simulink model "CM515A_MotAg4Meas"  (R2013b)
settings: Solver=VariableStepDiscrete  SolverMode=SingleTasking  StartTime=0.0  StopTime=1  FixedStep=0.002  RelTol=1e-3
values from neighbouring files (symbols this model uses):
  MOTAGCNTRREGMASK_CNT_U16 = DataDict.Constant    [CM515A_MotAg4Meas_DataDict.m]
  MOTAGLIM_CNT_U16 = DataDict.Constant    [CM515A_MotAg4Meas_DataDict.m]
undefined symbols (not defined in the file or in its folder): sigbuilder_block
libraries: simulink x4, NexteerUtilities x1
settings Model: RequirementInfo="{}  %GIDa_ca294f38_ed7c_4fb9_8c54_f4d56271bfc7"  ModifiedHistory=Rev 008: Updated model to Matlab 2013B, added comments to show requirement linkage  PauseTimes=0.5  Creator=nz3zln  LastModifiedBy=tzbsjd
settings SolverCC: AutoInsertRateTranBlk=on  InsertRTBMode=Always
settings DataIOCC: LimitDataPoints=off  SaveFormat=Structure  ReturnWorkspaceOutputs=on
settings OptimizationCC: BlockReduction=off  InlineParams=on  ZeroExternalMemoryAtStartup=off  ZeroInternalMemoryAtStartup=off  OptimizeModelRefInitCode=on  LifeSpan=1
settings DebuggingCC: SignalInfNanChecking=error  SignalRangeChecking=warning  UnderspecifiedInitializationDetection=Simplified  SolverPrmCheckMsg=error  InheritedTsInSrcMsg=error  DiscreteInheritContinuousMsg=error  SingleTaskRateTransMsg=error  TasksWithSamePriorityMsg=error  SigSpecEnsureSampleTimeMsg=error  CheckMatrixSingularityMsg=error  ParameterUnderflowMsg=error  ParameterPrecisionLossMsg=error  ParameterTunabilityLossMsg=error  FixptConstUnderflowMsg=warning  FixptConstOverflowMsg=warning  VectorMatrixConversionMsg=error  SignalLabelMismatchMsg=error  UnconnectedInputMsg=error  UnconnectedOutputMsg=error  UnconnectedLineMsg=error  SFcnCompatibilityMsg=error  UniqueDataStoreMsg=warning  BusObjectLabelMismatch=error  RootOutportRequireBusObject=error  AssertControl=DisableAll  ModelReferenceIOMsg=error  ModelReferenceVersionMismatchMessage=warning  ModelReferenceIOMismatchMessage=error  ModelReferenceCSMismatchMessage=warning  ModelReferenceDataLoggingMessage=error  StateNameClashWarn=warning  StrictBusMsg=ErrorOnBusTreatedAsVector  NonBusSignalsTreatedAsBus=error  SFUnexpectedBacktrackingDiag=error  SFInvalidInputDataAccessInChartInitDiag=error  SFNoUnconditionalDefaultTransitionDiag=error  SFTransitionOutsideNaturalParentDiag=error  SFUnconditionalTransitionShadowingDiag=error  SFUndirectedBroadcastEventsDiag=error
settings ModelReferenceCC: ModelReferenceNumInstancesAllowed=Single
settings RTWCC: SystemTargetFile=autosar.tlc  GenCodeOnly=on  TemplateMakefile=ert_default_tmf  Description=AUTOSAR  GenerateReport=on  ProcessScript=autosar_make_rtw_hook  LaunchReport=on
settings CodeAppCC: GenerateComments=off  IgnoreCustomStorageClasses=off  CustomSymbolStrType=$N$R$M  CustomSymbolStrBlkIO=$N$M  SimulinkBlockComments=off
settings STFCustomTargetCC: ParMdlRefBuildCompliant=on  CompOptLevelCompliant=on  IncludeMdlTerminateFcn=off  CombineOutputUpdateFcns=on  SuppressErrorStatus=on  ERTFirstTimeCompliant=on  ERTCustomFileBanners=on  SupportNonFinite=off  SupportComplex=off  SupportContinuousTime=off  SupportNonInlinedSFcns=off  MATLABClassNameForMDSCustomization=Simulink.SoftwareTarget.ERTCustomization  AutosarCompliant=on  GRTInterface=off  SystemTargetFile=autosar.tlc
settings ERTTargetCC: CodeReplacementLibrary=ANSI_C  ConcurrentExecutionCompliant=off  IncludeMdlTerminateFcn=off  SuppressErrorStatus=on  SupportNonFinite=off  SupportComplex=off  ModelStepFunctionPrototypeControlCompliant=off  CPPClassGenCompliant=off  AutosarCompliant=on  InlinedParameterPlacement=NonHierarchical  ERTCustomFileTemplate=example_file_process.tlc  EnableUserReplacementTypes=on

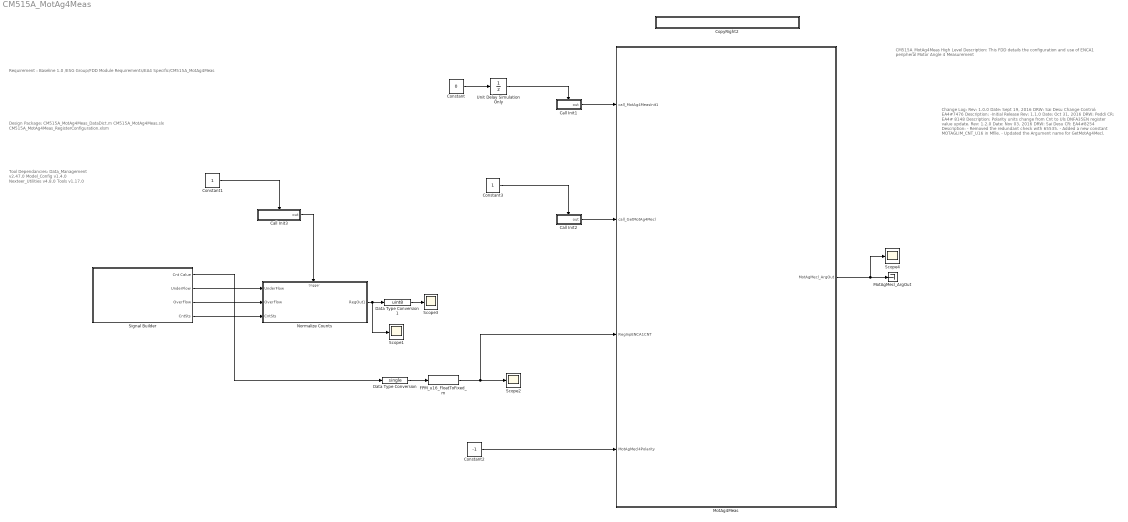
== system CM515A_MotAg4Meas ==
  note: Requirement : Baseline 1.0
      | /ESG Group/FDD Module Requirements/EA4 Specific/CM515A_MotAg4Meas
  note: Design Package:
      | CM515A_MotAg4Meas_DataDict.m
      | CM515A_MotAg4Meas.slx
      | CM515A_MotAg4Meas_RegisterConfiguration.xlsm
  note: CM515A_MotAg4Meas
      | High Level Description:
      | This FDD details the configuration and use of ENCA1 peripheral Motor Angle 4 Measurement
  note: Tool Dependancies:
      | Data_Management v2.47.0
      | Model_Config v1.4.0
      | Nexteer_Utilities v4.8.0
      | Tools v1.17.0
  note: Change Log:
      |
      | Rev: 1.0.0
      | Date: Sept 19, 2016
      | DRW: Sai Desu
      | Change Control: EA4#7476
      | Description:
      | -Initial Release
      |
      | Rev: 1.1.0
      | Date: Oct 31, 2016
      | DRW: Peddi
      | CR: EA4# 8148
      | Description: Polarity units change from Cnt to Uls
      | DNFA35EN register value update.
      |
      | Rev: 1.2.0
      | Date: Nov 03, 2016
      | DRW: Sai Desu
      | CR: EA4#8254
      | Description:
      | - Removed the redundant check with 65535.
      | - Added a new constant MOTAGLIM_CNT_U16 in  Mfile.
      | - Updated the Argument name for GetMotAg4Mecl.
  Call Init1 : Subsystem  TreatAsAtomicUnit=on
  Call Init2 : Subsystem  TreatAsAtomicUnit=on
  Call Init3 : Subsystem  TreatAsAtomicUnit=on
  Constant : Constant  Value=0  OutDataTypeStr=uint8
  Constant1 : Constant  OutDataTypeStr=int8
  Constant2 : Constant  Value=-1  OutDataTypeStr=int8
  Constant3 : Constant  OutDataTypeStr=int8
  CopyRight2 : Subsystem  Description=|  mask(Copyright Information){none=on}
      | Copyright info block.                                               
      |                                                                     
      | Place copyright information at the top of every subsystem in design.
      mask prompts: none "No parameters"
      mask help: Place copyright information at the top of every subsystem in design.
      mask Display:
      | NxtrConf = 'Nexteer Confidential';
      | 
      | sys = bdroot; %handle for the current model ("system")
      | first = get_param(sys,'Created');
      | first = first(end-3:end);  %year is last four digits
      | 
      | last = get_param(sys,'LastModifiedDate');
      | if isempty(last)
      |     last = datestr(now,'yyyy');
      | else
      |     last = last(end-3:end);
      | end
      | 
      | if strcmp(first,last)
      |     fprintf('%s -- Copyright %s Nexteer',NxtrConf,first)
      | else
      |     fprintf('%s -- %s%s- %s Nexteer',NxtrConf,char(169),first,last)
      | end
  Data Type Conversion : DataTypeConversion  OutDataTypeStr=single
  Data Type Conversion1 : DataTypeConversion  OutDataTypeStr=uint8
  FPM_u16_FloatToFixed_m : NexteerUtilities/Fixed Point Math Conversions/FPM_u16_FloatToFixed_m  SFunctionSpec=uint16 y1 = FPM_u16_FloatToFixed_m(single u1, single p1)  Param1=16
      settings: AttributesFormatString=u16_FloatToFixed
  MotAg4Meas : Subsystem
  MotAgMecl_ArgOut : Terminator
  Normalize Counts : Subsystem
  Scope{1..4} (4 alike) : Scope
      Scope2 settings: SaveName=ScopeData7
      Scope4 settings: SaveName=ScopeData2
  Signal Builder : Subsystem  Tag=STV Subsys  LoadFcn=sigbuilder_block('load');  StartFcn=sigbuilder_block('start');  StopFcn=sigbuilder_block('stop');  ClipboardFcn=sigbuilder_block('clipboard');  mask(Sigbuilder block){}
      mask help: Simulink:masks:SigbuilderBlock_MD
      mask init:
      | if ~strcmp(get_param(bdroot(gcbh),'SimulationStatus'),'stopped') tuvar = sigbuilder_block('maskInit'); end
      settings: CopyFcn=sigbuilder_block('copy');  DeleteFcn=sigbuilder_block('delete');  ModelCloseFcn=sigbuilder_block('modelClose');  PreSaveFcn=sigbuilder_block('preSave');  PauseFcn=sigbuilder_block('pause');  ContinueFcn=sigbuilder_block('continue');  NameChangeFcn=sigbuilder_block('namechange');  OpenFcn=sigbuilder_block('open',[0 30 1440 723 ]);  CloseFcn=sigbuilder_block('close');
      mask Display: plot(0, 0, 100, 100,[2, 2, 32, 32, 2], [68, 8, 8, 68, 68],[32, 2], [38, 38], [32, 19, 2],[53, 60, 44], [32, 17, 17, 2],[16, 16, 31, 31]);txt = getActiveGroup(gcbh);text(2, 100, txt,'verticalAlignment', 'top');
  Unit Delay Simulation Only : UnitDelay  InitialCondition=1  SampleTime=-1
  wires:
  Constant/1 -> Unit Delay Simulation Only/1
  Unit Delay Simulation Only/1 -> Call Init1/Enable
  Constant3/1 -> Call Init2/Enable
  Call Init1/1(out) -> MotAg4Meas/1(call_MotAg4MeasInit1)
  Call Init2/1(out) -> MotAg4Meas/2(call_GetMotAg4Mecl)
  FPM_u16_FloatToFixed_m/1 -> MotAg4Meas/3(RegInpENCA1CNT), Scope2/1
  Normalize Counts/1(RegOut1) -> Data Type Conversion1/1, Scope1/1
  MotAg4Meas/1(MotAgMecl_ArgOut) -> Scope4/1, MotAgMecl_ArgOut/1
  Data Type Conversion/1 -> FPM_u16_FloatToFixed_m/1
  Constant1/1 -> Call Init3/Enable
  Call Init3/1(out) -> Normalize Counts/Trigger
  Signal Builder/1(Cnt Calue) -> Data Type Conversion/1
  Signal Builder/2(UnderFlow) -> Normalize Counts/1(UnderFlow)
  Signal Builder/3(OverFlow) -> Normalize Counts/2(OverFlow)
  Signal Builder/4(CntSts) -> Normalize Counts/3(CntSts)
  Data Type Conversion1/1 -> Scope3/1
  Constant2/1 -> MotAg4Meas/4(MotAgMecl4Polarity)

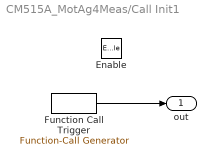
== system CM515A_MotAg4Meas/Call Init1 ==
  Enable : EnablePort
  Function Call Trigger : simulink/Ports & Subsystems/Function-Call Generator  RequirementInfo={} %GIDa_b7229461_487a_40de_bfdf_dab388053d82  sample_time=0.002  numberOfIterations=1
  out : Outport
  wires:
  Function Call Trigger/1 -> out/1

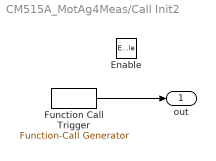
== system CM515A_MotAg4Meas/Call Init2 ==
  Enable : EnablePort
  Function Call Trigger : simulink/Ports & Subsystems/Function-Call Generator  RequirementInfo={} %GIDa_a0a97c4f_3e8f_431b_a781_191ff84f73ef  sample_time=0.0005  numberOfIterations=1
  out : Outport
  wires:
  Function Call Trigger/1 -> out/1

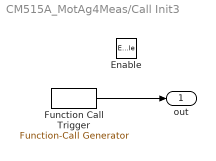
== system CM515A_MotAg4Meas/Call Init3 ==
  Enable : EnablePort
  Function Call Trigger : simulink/Ports & Subsystems/Function-Call Generator  RequirementInfo={} %GIDa_a0a97c4f_3e8f_431b_a781_191ff84f73ef  sample_time=0.0005  numberOfIterations=1
  out : Outport
  wires:
  Function Call Trigger/1 -> out/1

== system CM515A_MotAg4Meas/CopyRight2 ==

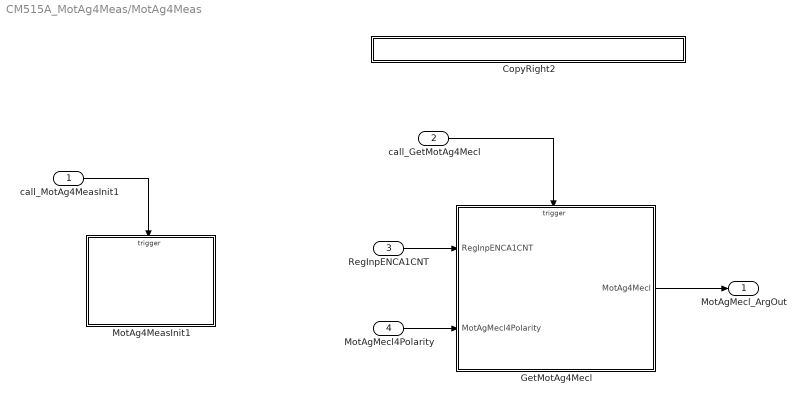
== system CM515A_MotAg4Meas/MotAg4Meas ==
  call_MotAg4MeasInit1 : Inport  RequirementInfo={} %GIDa_3f2124e9_01f6_42c8_98ca_c09f4c17d99d
  call_GetMotAg4Mecl : Inport  RequirementInfo={} %GIDa_a9829b41_47bf_4b01_8e96_1bb4faec4565  Port=2
  RegInpENCA1CNT : Inport  Port=3
  MotAgMecl4Polarity : Inport  Port=4
  CopyRight2 : Subsystem  Description=|  mask(Copyright Information){none=on}
      | Copyright info block.                                               
      |                                                                     
      | Place copyright information at the top of every subsystem in design.
      mask prompts: none "No parameters"
      mask help: Place copyright information at the top of every subsystem in design.
      mask Display:
      | NxtrConf = 'Nexteer Confidential';
      | 
      | sys = bdroot; %handle for the current model ("system")
      | first = get_param(sys,'Created');
      | first = first(end-3:end);  %year is last four digits
      | 
      | last = get_param(sys,'LastModifiedDate');
      | if isempty(last)
      |     last = datestr(now,'yyyy');
      | else
      |     last = last(end-3:end);
      | end
      | 
      | if strcmp(first,last)
      |     fprintf('%s -- Copyright %s Nexteer',NxtrConf,first)
      | else
      |     fprintf('%s -- %s%s- %s Nexteer',NxtrConf,char(169),first,last)
      | end
  GetMotAg4Mecl : Subsystem  RequirementInfo={} %GIDa_dbd08618_b447_4b13_a314_37af3685d10a
  MotAg4MeasInit1 : Subsystem
  MotAgMecl_ArgOut : Outport
  wires:
  call_MotAg4MeasInit1/1 -> MotAg4MeasInit1/Trigger
  call_GetMotAg4Mecl/1 -> GetMotAg4Mecl/Trigger
  RegInpENCA1CNT/1 -> GetMotAg4Mecl/1(RegInpENCA1CNT)
  GetMotAg4Mecl/1(MotAg4Mecl) -> MotAgMecl_ArgOut/1
  MotAgMecl4Polarity/1 -> GetMotAg4Mecl/2(MotAgMecl4Polarity)

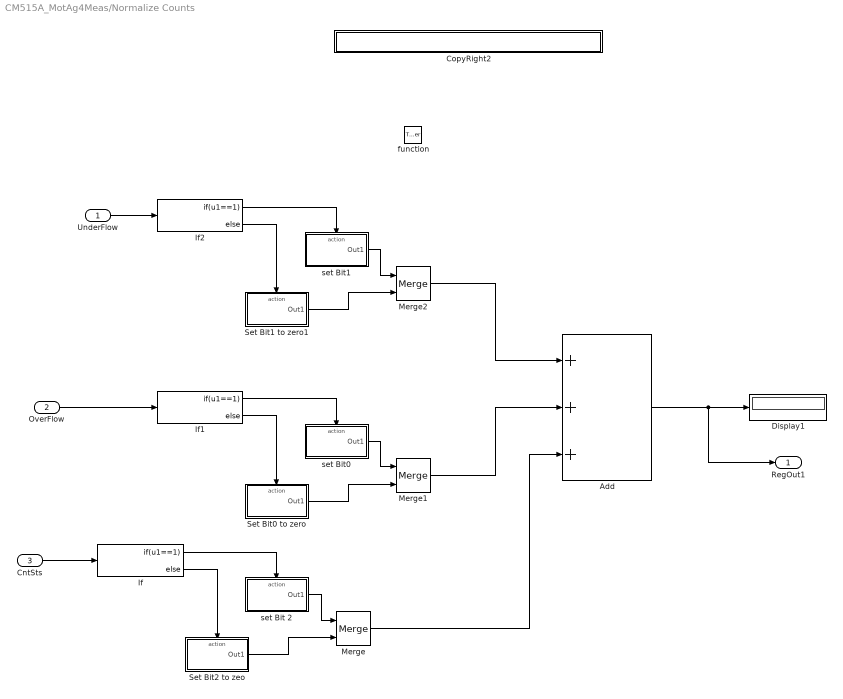
== system CM515A_MotAg4Meas/Normalize Counts ==
  UnderFlow : Inport
  OverFlow : Inport  Port=2
  CntSts : Inport  Port=3
  function : TriggerPort  TriggerType=function-call
  Add : Sum  Inputs=+++
  CopyRight2 : Subsystem  Description=|  mask(Copyright Information){none=on}
      | Copyright info block.                                               
      |                                                                     
      | Place copyright information at the top of every subsystem in design.
      mask prompts: none "No parameters"
      mask help: Place copyright information at the top of every subsystem in design.
      mask Display:
      | NxtrConf = 'Nexteer Confidential';
      | 
      | sys = bdroot; %handle for the current model ("system")
      | first = get_param(sys,'Created');
      | first = first(end-3:end);  %year is last four digits
      | 
      | last = get_param(sys,'LastModifiedDate');
      | if isempty(last)
      |     last = datestr(now,'yyyy');
      | else
      |     last = last(end-3:end);
      | end
      | 
      | if strcmp(first,last)
      |     fprintf('%s -- Copyright %s Nexteer',NxtrConf,first)
      | else
      |     fprintf('%s -- %s%s- %s Nexteer',NxtrConf,char(169),first,last)
      | end
  Display1 : Display
  If : If  IfExpression=u1==1
  If1 : If  IfExpression=u1==1
  If2 : If  IfExpression=u1==1
  Merge : Merge
  Merge1 : Merge
  Merge2 : Merge
  Set Bit0 to zero : Subsystem  TreatAsAtomicUnit=on
  Set Bit1 to zero1 : Subsystem  TreatAsAtomicUnit=on
  Set Bit2 to zeo : Subsystem  TreatAsAtomicUnit=on
  set Bit 2 : Subsystem  TreatAsAtomicUnit=on
  set Bit0 : Subsystem  TreatAsAtomicUnit=on
  set Bit1 : Subsystem  TreatAsAtomicUnit=on
  RegOut1 : Outport
  wires:
  CntSts/1 -> If/1
  If/1 -> set Bit 2/Action
  If/2 -> Set Bit2 to zeo/Action
  set Bit 2/1(Out1) -> Merge/1
  Set Bit2 to zeo/1(Out1) -> Merge/2
  If1/1 -> set Bit0/Action
  If1/2 -> Set Bit0 to zero/Action
  set Bit0/1(Out1) -> Merge1/1
  Set Bit0 to zero/1(Out1) -> Merge1/2
  OverFlow/1 -> If1/1
  If2/1 -> set Bit1/Action
  If2/2 -> Set Bit1 to zero1/Action
  set Bit1/1(Out1) -> Merge2/1
  Set Bit1 to zero1/1(Out1) -> Merge2/2
  UnderFlow/1 -> If2/1
  Merge2/1 -> Add/1
  Merge1/1 -> Add/2
  Merge/1 -> Add/3
  Add/1 -> RegOut1/1, Display1/1

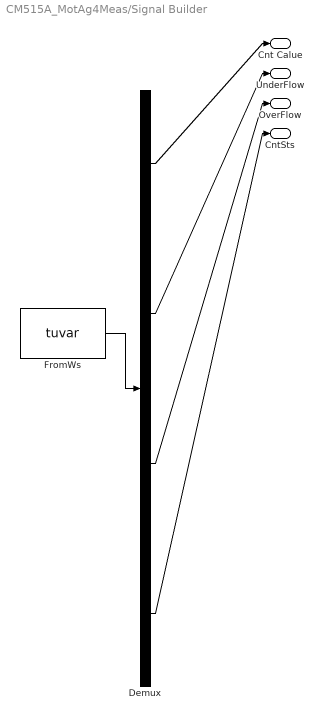
== system CM515A_MotAg4Meas/Signal Builder ==
  Demux : Demux  Tag=STV Demux
  FromWs : FromWorkspace  Tag=STV FromWs  VariableName=tuvar  SampleTime=0
      SigBuilderData=|
      | common.afterFinalStr = 'Extrapolate'
      | common.sampleTime = 0
      | dataSet(1).timeRange = [0 1]
      | dataSet(1).name = 'UpCount'
      | dataSet(2).timeRange = [0 1]
      | dataSet(2).name = 'DownCount'
      | sbobj.Groups(1).Name = 'UpCount'
      | sbobj.Groups(1).Signals(1).Name = 'Cnt Calue'
      | sbobj.Groups(1).Signals(1).XData = [0 0.2 0.2 0.3 0.4 0.4 0.6 1]
      | sbobj.Groups(1).Signals(1).YData = [0 1 0 0.5 0 1 0 1]
      | sbobj.Groups(1).Signals(2).Name = 'UnderFlow'
      | sbobj.Groups(1).Signals(2).XData = [0 0.5 1]
      | sbobj.Groups(1).Signals(2).YData = [0 0 0]
      | sbobj.Groups(1).Signals(3).Name = 'OverFlow'
      | sbobj.Groups(1).Signals(3).XData = [0 0.499 0.499 0.5 0.5 1]
      | sbobj.Groups(1).Signals(3).YData = [0 0 1 1 0 0]
      | sbobj.Groups(1).Signals(4).Name = 'CntSts'
      | sbobj.Groups(1).Signals(4).XData = [0 1]
      | sbobj.Groups(1).Signals(4).YData = [0 0]
      | sbobj.Groups(1).TimeRange = [0 1]
      | sbobj.Groups(2).Name = 'DownCount'
      | sbobj.Groups(2).Signals(1).Name = 'Cnt Calue'
      | sbobj.Groups(2).Signals(1).XData = [0 1]
      | sbobj.Groups(2).Signals(1).YData = [1 0]
      | sbobj.Groups(2).Signals(2).Name = 'UnderFlow'
      | sbobj.Groups(2).Signals(2).XData = [0 0.499 0.499 0.5 0.5 1]
      | sbobj.Groups(2).Signals(2).YData = [0 0 1 1 0 0]
      | sbobj.Groups(2).Signals(3).Name = 'OverFlow'
      | sbobj.Groups(2).Signals(3).XData = [0 1]
      | sbobj.Groups(2).Signals(3).YData = [0 0]
      | sbobj.Groups(2).Signals(4).Name = 'CntSts'
      | sbobj.Groups(2).Signals(4).XData = [0 1]
      | sbobj.Groups(2).Signals(4).YData = [1 1]
      | sbobj.Groups(2).TimeRange = [0 1]
  Cnt Calue : Outport  Tag=STV Outport
  UnderFlow : Outport  Tag=STV Outport  Port=2
  OverFlow : Outport  Tag=STV Outport  Port=3
  CntSts : Outport  Tag=STV Outport  Port=4
  wires:
  FromWs/1 -> Demux/1
  Demux/1 -> Cnt Calue/1
  Demux/2 -> UnderFlow/1
  Demux/3 -> OverFlow/1
  Demux/4 -> CntSts/1

== system CM515A_MotAg4Meas/MotAg4Meas/CopyRight2 ==

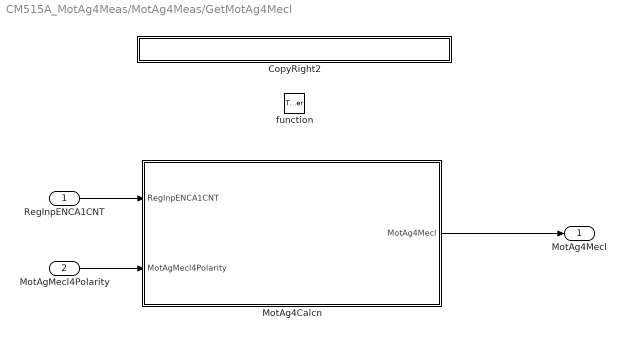
== system CM515A_MotAg4Meas/MotAg4Meas/GetMotAg4Mecl ==
  RegInpENCA1CNT : Inport
  MotAgMecl4Polarity : Inport  Port=2
  function : TriggerPort  TriggerType=function-call
  CopyRight2 : Subsystem  Description=|  mask(Copyright Information){none=on}
      | Copyright info block.                                               
      |                                                                     
      | Place copyright information at the top of every subsystem in design.
      mask prompts: none "No parameters"
      mask help: Place copyright information at the top of every subsystem in design.
      mask Display:
      | NxtrConf = 'Nexteer Confidential';
      | 
      | sys = bdroot; %handle for the current model ("system")
      | first = get_param(sys,'Created');
      | first = first(end-3:end);  %year is last four digits
      | 
      | last = get_param(sys,'LastModifiedDate');
      | if isempty(last)
      |     last = datestr(now,'yyyy');
      | else
      |     last = last(end-3:end);
      | end
      | 
      | if strcmp(first,last)
      |     fprintf('%s -- Copyright %s Nexteer',NxtrConf,first)
      | else
      |     fprintf('%s -- %s%s- %s Nexteer',NxtrConf,char(169),first,last)
      | end
  MotAg4Calcn : Subsystem  RequirementInfo="{'linktype_rmi_doors' '00011b55 (/ESG Group/FDD Module Requirements/EA4 Specific/CM515A_MotAg4Meas)' '#CM515A_15' 'true' 'REQ:  CM515A_15' '' } %GIDa_14b6ebf1_d9a3_430c_bf27_c6bb9d0b9ccf"
  MotAg4Mecl : Outport
  wires:
  RegInpENCA1CNT/1 -> MotAg4Calcn/1(RegInpENCA1CNT)
  MotAg4Calcn/1(MotAg4Mecl) -> MotAg4Mecl/1
  MotAgMecl4Polarity/1 -> MotAg4Calcn/2(MotAgMecl4Polarity)

== system CM515A_MotAg4Meas/MotAg4Meas/MotAg4MeasInit1 ==
  function : TriggerPort  TriggerType=function-call
  CopyRight2 : Subsystem  Description=|  mask(Copyright Information){none=on}
      | Copyright info block.                                               
      |                                                                     
      | Place copyright information at the top of every subsystem in design.
      mask prompts: none "No parameters"
      mask help: Place copyright information at the top of every subsystem in design.
      mask Display:
      | NxtrConf = 'Nexteer Confidential';
      | 
      | sys = bdroot; %handle for the current model ("system")
      | first = get_param(sys,'Created');
      | first = first(end-3:end);  %year is last four digits
      | 
      | last = get_param(sys,'LastModifiedDate');
      | if isempty(last)
      |     last = datestr(now,'yyyy');
      | else
      |     last = last(end-3:end);
      | end
      | 
      | if strcmp(first,last)
      |     fprintf('%s -- Copyright %s Nexteer',NxtrConf,first)
      | else
      |     fprintf('%s -- %s%s- %s Nexteer',NxtrConf,char(169),first,last)
      | end
  Initialize ENCA Registers : Subsystem  TreatAsAtomicUnit=on

== system CM515A_MotAg4Meas/Normalize Counts/CopyRight2 ==

== system CM515A_MotAg4Meas/Normalize Counts/Set Bit0 to zero ==
  Action Port : ActionPort  ActionType=else
  Constant : Constant  Value=0  OutDataTypeStr=uint8
  Out1 : Outport
  wires:
  Constant/1 -> Out1/1

== system CM515A_MotAg4Meas/Normalize Counts/Set Bit1 to zero1 ==
  Action Port : ActionPort  ActionType=else
  Constant : Constant  Value=0  OutDataTypeStr=uint8
  Out1 : Outport
  wires:
  Constant/1 -> Out1/1

== system CM515A_MotAg4Meas/Normalize Counts/Set Bit2 to zeo ==
  Action Port : ActionPort  ActionType=else
  Constant : Constant  Value=0  OutDataTypeStr=uint8
  Out1 : Outport
  wires:
  Constant/1 -> Out1/1

== system CM515A_MotAg4Meas/Normalize Counts/set Bit 2 ==
  Action Port : ActionPort  ActionType=then
  Constant : Constant  Value=4  OutDataTypeStr=uint8
  Out1 : Outport
  wires:
  Constant/1 -> Out1/1

== system CM515A_MotAg4Meas/Normalize Counts/set Bit0 ==
  Action Port : ActionPort  ActionType=then
  Constant : Constant  OutDataTypeStr=uint8
  Out1 : Outport
  wires:
  Constant/1 -> Out1/1

== system CM515A_MotAg4Meas/Normalize Counts/set Bit1 ==
  Action Port : ActionPort  ActionType=then
  Constant : Constant  Value=2  OutDataTypeStr=uint8
  Out1 : Outport
  wires:
  Constant/1 -> Out1/1

== system CM515A_MotAg4Meas/MotAg4Meas/GetMotAg4Mecl/CopyRight2 ==

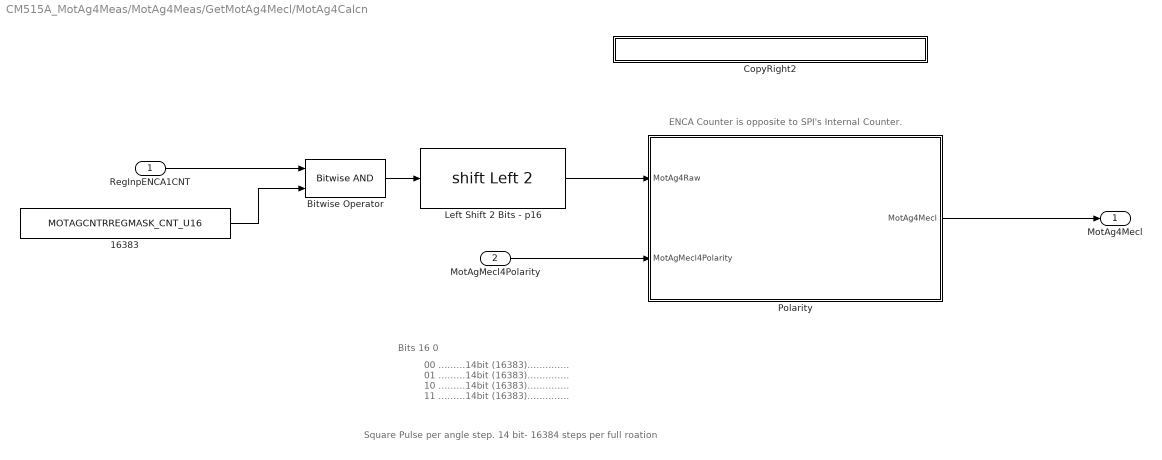
== system CM515A_MotAg4Meas/MotAg4Meas/GetMotAg4Mecl/MotAg4Calcn ==
  note: Square Pulse per angle step. 14 bit- 16384 steps per full roation
  note: ENCA Counter is opposite to SPI's Internal Counter.
  note: Bits 16 0
  note: 00 .........14bit (16383)..............
      | 01 .........14bit (16383)..............
      | 10 .........14bit (16383)..............
      | 11 .........14bit (16383)..............
  RegInpENCA1CNT : Inport  RequirementInfo="{'linktype_rmi_doors' '00011b55 (/ESG Group/FDD Module Requirements/EA4 Specific/CM515A_MotAg4Meas)' '#CM515A_66' 'true' 'REQ:  CM515A_66' '' } %GIDa_08ec8d51_6bf0_485e_bf0c_e07448ca5708"
  MotAgMecl4Polarity : Inport  RequirementInfo={} %GIDa_a154c5c1_f9bb_4438_a4db_c13dbdf13071  Port=2
  16383 : Constant  RequirementInfo="{'linktype_rmi_doors' '00011b55 (/ESG Group/FDD Module Requirements/EA4 Specific/CM515A_MotAg4Meas)' '#CM515A_66' 'true' 'REQ:  CM515A_66' '' } %GIDa_c0dd3f32_81e1_4d09_b8fe_2e8838c8b21c"  Value=MOTAGCNTRREGMASK_CNT_U16
  Bitwise Operator : simulink/Logic and Bit Operations/Bitwise Operator  RequirementInfo="{'linktype_rmi_doors' '00011b55 (/ESG Group/FDD Module Requirements/EA4 Specific/CM515A_MotAg4Meas)' '#CM515A_66' 'true' 'REQ:  CM515A_66' '' } %GIDa_a2bf002a_d1f5_43d9_b1cc_8ae2bafc417c"  logicop=AND  UseBitMask=off  NumInputPorts=2  BitMask=16383  BitMaskRealWorld=Stored Integer
  CopyRight2 : Subsystem  Description=|  mask(Copyright Information){none=on}
      | Copyright info block.                                               
      |                                                                     
      | Place copyright information at the top of every subsystem in design.
      mask prompts: none "No parameters"
      mask help: Place copyright information at the top of every subsystem in design.
      mask Display:
      | NxtrConf = 'Nexteer Confidential';
      | 
      | sys = bdroot; %handle for the current model ("system")
      | first = get_param(sys,'Created');
      | first = first(end-3:end);  %year is last four digits
      | 
      | last = get_param(sys,'LastModifiedDate');
      | if isempty(last)
      |     last = datestr(now,'yyyy');
      | else
      |     last = last(end-3:end);
      | end
      | 
      | if strcmp(first,last)
      |     fprintf('%s -- Copyright %s Nexteer',NxtrConf,first)
      | else
      |     fprintf('%s -- %s%s- %s Nexteer',NxtrConf,char(169),first,last)
      | end
  Left Shift 2 Bits - p16 : ArithShift  RequirementInfo="{'linktype_rmi_doors' '00011b55 (/ESG Group/FDD Module Requirements/EA4 Specific/CM515A_MotAg4Meas)' '#CM515A_66' 'true' 'REQ:  CM515A_66' '' } %GIDa_e6c89e43_3576_4000_a35f_842f25e1a1b7"  BitShiftNumber=2  BitShiftDirection=Left
  Polarity : Subsystem  RequirementInfo="{'linktype_rmi_doors' '00011b55 (/ESG Group/FDD Module Requirements/EA4 Specific/CM515A_MotAg4Meas)' '#CM515A_67' 'true' 'REQ:  CM515A_67' '' } %GIDa_f744dcfa_c060_4788_aa5c_dd845431b195"
  MotAg4Mecl : Outport
  wires:
  Polarity/1(MotAg4Mecl) -> MotAg4Mecl/1
  Bitwise Operator/1 -> Left Shift 2 Bits - p16/1
  Left Shift 2 Bits - p16/1 -> Polarity/1(MotAg4Raw)
  RegInpENCA1CNT/1 -> Bitwise Operator/1
  16383/1 -> Bitwise Operator/2
  MotAgMecl4Polarity/1 -> Polarity/2(MotAgMecl4Polarity)

== system CM515A_MotAg4Meas/MotAg4Meas/MotAg4MeasInit1/CopyRight2 ==

== system CM515A_MotAg4Meas/MotAg4Meas/MotAg4MeasInit1/Initialize ENCA Registers ==
  note: Configure the ENCA registers according to CM515A_MotAg4Meas_RegisterConfiguration.xlsm
      |     Order by Row.
  CopyRight2 : Subsystem  Description=|  mask(Copyright Information){none=on}
      | Copyright info block.                                               
      |                                                                     
      | Place copyright information at the top of every subsystem in design.
      mask prompts: none "No parameters"
      mask help: Place copyright information at the top of every subsystem in design.
      mask Display:
      | NxtrConf = 'Nexteer Confidential';
      | 
      | sys = bdroot; %handle for the current model ("system")
      | first = get_param(sys,'Created');
      | first = first(end-3:end);  %year is last four digits
      | 
      | last = get_param(sys,'LastModifiedDate');
      | if isempty(last)
      |     last = datestr(now,'yyyy');
      | else
      |     last = last(end-3:end);
      | end
      | 
      | if strcmp(first,last)
      |     fprintf('%s -- Copyright %s Nexteer',NxtrConf,first)
      | else
      |     fprintf('%s -- %s%s- %s Nexteer',NxtrConf,char(169),first,last)
      | end

== system CM515A_MotAg4Meas/MotAg4Meas/GetMotAg4Mecl/MotAg4Calcn/CopyRight2 ==

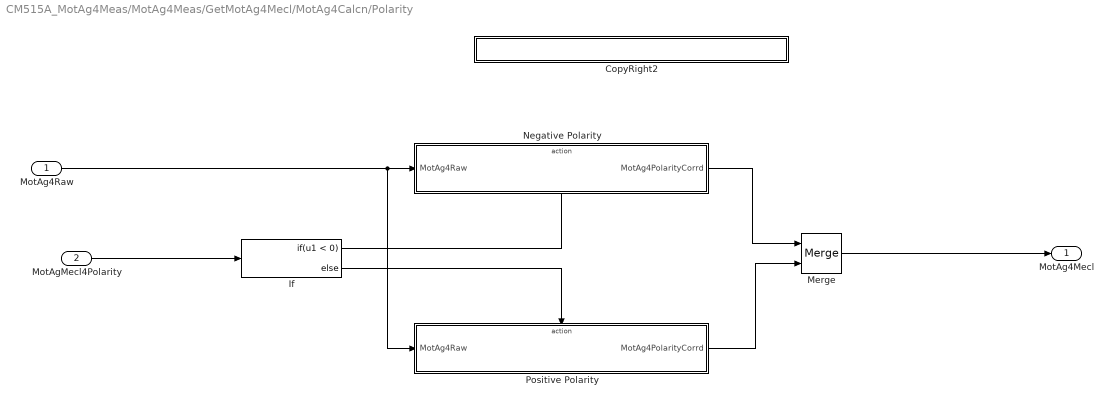
== system CM515A_MotAg4Meas/MotAg4Meas/GetMotAg4Mecl/MotAg4Calcn/Polarity ==
  MotAg4Raw : Inport
  MotAgMecl4Polarity : Inport  Port=2
  CopyRight2 : Subsystem  Description=|  mask(Copyright Information){none=on}
      | Copyright info block.                                               
      |                                                                     
      | Place copyright information at the top of every subsystem in design.
      mask prompts: none "No parameters"
      mask help: Place copyright information at the top of every subsystem in design.
      mask Display:
      | NxtrConf = 'Nexteer Confidential';
      | 
      | sys = bdroot; %handle for the current model ("system")
      | first = get_param(sys,'Created');
      | first = first(end-3:end);  %year is last four digits
      | 
      | last = get_param(sys,'LastModifiedDate');
      | if isempty(last)
      |     last = datestr(now,'yyyy');
      | else
      |     last = last(end-3:end);
      | end
      | 
      | if strcmp(first,last)
      |     fprintf('%s -- Copyright %s Nexteer',NxtrConf,first)
      | else
      |     fprintf('%s -- %s%s- %s Nexteer',NxtrConf,char(169),first,last)
      | end
  If : If  IfExpression=u1 < 0
  Merge : Merge
  Negative Polarity : Subsystem  TreatAsAtomicUnit=on
  Positive Polarity : Subsystem  TreatAsAtomicUnit=on
  MotAg4Mecl : Outport
  wires:
  MotAgMecl4Polarity/1 -> If/1
  MotAg4Raw/1 -> Positive Polarity/1(MotAg4Raw), Negative Polarity/1(MotAg4Raw)
  If/1 -> Negative Polarity/Action
  If/2 -> Positive Polarity/Action
  Negative Polarity/1(MotAg4PolarityCorrd) -> Merge/1
  Positive Polarity/1(MotAg4PolarityCorrd) -> Merge/2
  Merge/1 -> MotAg4Mecl/1

== system CM515A_MotAg4Meas/MotAg4Meas/MotAg4MeasInit1/Initialize ENCA Registers/CopyRight2 ==

== system CM515A_MotAg4Meas/MotAg4Meas/GetMotAg4Mecl/MotAg4Calcn/Polarity/CopyRight2 ==

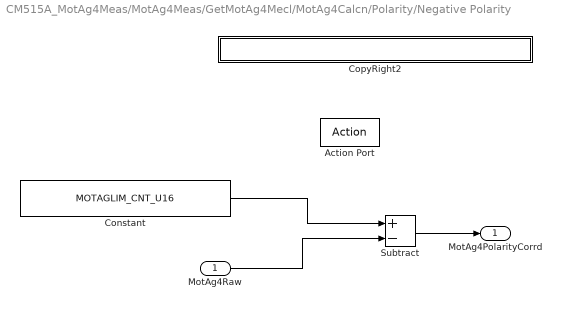
== system CM515A_MotAg4Meas/MotAg4Meas/GetMotAg4Mecl/MotAg4Calcn/Polarity/Negative Polarity ==
  MotAg4Raw : Inport
  Action Port : ActionPort  ActionType=then
  Constant : Constant  Value=MOTAGLIM_CNT_U16
  CopyRight2 : Subsystem  Description=|  mask(Copyright Information){none=on}
      | Copyright info block.                                               
      |                                                                     
      | Place copyright information at the top of every subsystem in design.
      mask prompts: none "No parameters"
      mask help: Place copyright information at the top of every subsystem in design.
      mask Display:
      | NxtrConf = 'Nexteer Confidential';
      | 
      | sys = bdroot; %handle for the current model ("system")
      | first = get_param(sys,'Created');
      | first = first(end-3:end);  %year is last four digits
      | 
      | last = get_param(sys,'LastModifiedDate');
      | if isempty(last)
      |     last = datestr(now,'yyyy');
      | else
      |     last = last(end-3:end);
      | end
      | 
      | if strcmp(first,last)
      |     fprintf('%s -- Copyright %s Nexteer',NxtrConf,first)
      | else
      |     fprintf('%s -- %s%s- %s Nexteer',NxtrConf,char(169),first,last)
      | end
  Subtract : Sum  Inputs=+-
  MotAg4PolarityCorrd : Outport
  wires:
  Constant/1 -> Subtract/1
  MotAg4Raw/1 -> Subtract/2
  Subtract/1 -> MotAg4PolarityCorrd/1

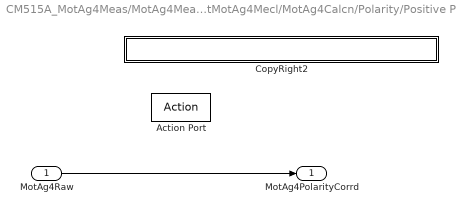
== system CM515A_MotAg4Meas/MotAg4Meas/GetMotAg4Mecl/MotAg4Calcn/Polarity/Positive Polarity ==
  MotAg4Raw : Inport
  Action Port : ActionPort  ActionType=else
  CopyRight2 : Subsystem  Description=|  mask(Copyright Information){none=on}
      | Copyright info block.                                               
      |                                                                     
      | Place copyright information at the top of every subsystem in design.
      mask prompts: none "No parameters"
      mask help: Place copyright information at the top of every subsystem in design.
      mask Display:
      | NxtrConf = 'Nexteer Confidential';
      | 
      | sys = bdroot; %handle for the current model ("system")
      | first = get_param(sys,'Created');
      | first = first(end-3:end);  %year is last four digits
      | 
      | last = get_param(sys,'LastModifiedDate');
      | if isempty(last)
      |     last = datestr(now,'yyyy');
      | else
      |     last = last(end-3:end);
      | end
      | 
      | if strcmp(first,last)
      |     fprintf('%s -- Copyright %s Nexteer',NxtrConf,first)
      | else
      |     fprintf('%s -- %s%s- %s Nexteer',NxtrConf,char(169),first,last)
      | end
  MotAg4PolarityCorrd : Outport
  wires:
  MotAg4Raw/1 -> MotAg4PolarityCorrd/1

== system CM515A_MotAg4Meas/MotAg4Meas/GetMotAg4Mecl/MotAg4Calcn/Polarity/Negative Polarity/CopyRight2 ==

== system CM515A_MotAg4Meas/MotAg4Meas/GetMotAg4Mecl/MotAg4Calcn/Polarity/Positive Polarity/CopyRight2 ==
